simulink model "testMdl"  (R2022b)
settings: Solver=VariableStepAuto  StartTime=0.0  StopTime=10.0  RelTol=1e-3
undefined symbols (not defined in the file or in its folder): mySLPart
settings Model: Creator=grouleau  LastModifiedBy=grouleau

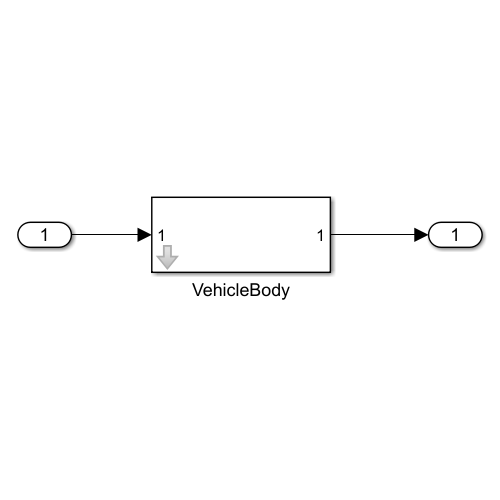
[thumbnail: Simulink's stored preview of the top-level diagram]
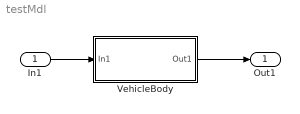
== system testMdl ==
  In1 : Inport
  VehicleBody : Subsystem  mask(Simulink Variant Part){obj=mySLPart}
      mask prompts: obj "Variant Part Object:"
  Out1 : Outport
  wires:
  In1/1 -> VehicleBody/1(In1)
  VehicleBody/1(Out1) -> Out1/1

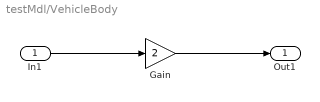
== system testMdl/VehicleBody ==
  In1 : Inport
  Gain : Gain  Gain=2
  Out1 : Outport
  wires:
  In1/1 -> Gain/1
  Gain/1 -> Out1/1
